simulink model "PID_controller_sim"  (R2021a)
settings: Solver=VariableStepAuto  StartTime=0.0  StopTime=inf  RelTol=1e-3
settings Model: Creator=bascetta  LastModifiedBy=bascetta
settings DataIOCC: FinalStateName=PID_controller_simSimState  SaveFinalState=on  SaveOperatingPoint=on  SaveOutput=off  SignalLogging=off  DSMLogging=off  SaveTime=off  ReturnWorkspaceOutputs=off

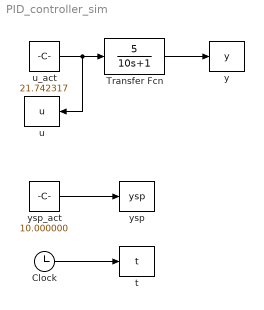
== system PID_controller_sim ==
  Clock : Clock
  Transfer Fcn : TransferFcn  Numerator=[5]  Denominator=[10 1]
  t : ToWorkspace  VariableName=t  SampleTime=0.010000
      settings: Save2DSignal=2-D array (concatenate along first dimension)
  u : ToWorkspace  VariableName=u  SampleTime=0.010000
      settings: Save2DSignal=2-D array (concatenate along first dimension)
  u_act : Constant  Value=21.742317
  y : ToWorkspace  VariableName=y  SampleTime=0.010000
      settings: Save2DSignal=2-D array (concatenate along first dimension)
  ysp : ToWorkspace  VariableName=ysp  SampleTime=0.010000
      settings: Save2DSignal=2-D array (concatenate along first dimension)
  ysp_act : Constant  Value=10.000000
  wires:
  u_act/1 -> u/1, Transfer Fcn/1
  Transfer Fcn/1 -> y/1
  ysp_act/1 -> ysp/1
  Clock/1 -> t/1
